simulink model "powerwindow_tl_v04"  (R2020b)
settings: Solver=ode1  StartTime=0.0  StopTime=20.0  FixedStep=0.01  RelTol=1e-3
PreLoadFcn:
  | if exist('tl_preloadfcn','file'), tl_preloadfcn(gcs,'5.1.0.29'); end
PostLoadFcn:
  | if exist('tl_postloadfcn','file'), tl_postloadfcn(gcs,'5.1.0.29'); end
InitFcn:
  | if exist('tlds_init','file'), tlds_init(gcs); end
StartFcn:
  | if exist('tlds_start','file'), tlds_start(gcs); end
StopFcn:
  | if exist('tlds_stop','file'), tlds_stop(gcs); end
undefined symbols (not defined in the file): auto_down_time, auto_up_time, emergency_down_time, position_endstop_top
libraries: tllib x7
(part 2 of 2)

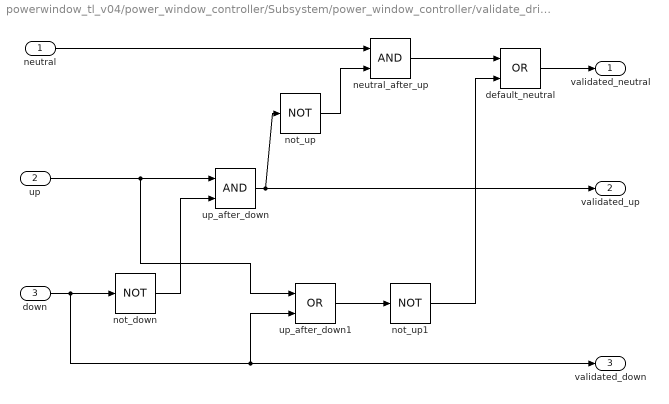
== system powerwindow_tl_v04/power_window_controller/Subsystem/power_window_controller/validate_driver/mutually_exclusive ==
  neutral : Inport  RequirementInfo={} %GIDa_e85989e4_f574_4415_bd99_a29a617e3f19
  up : Inport  RequirementInfo={} %GIDa_79e0b872_de73_4653_8aed_1078f22e8307  Port=2
  down : Inport  RequirementInfo={} %GIDa_e828e409_7827_4f1e_bdb2_ab00d1d51755  Port=3
  default_neutral : Logic  RequirementInfo={} %GIDa_6e7c89da_e8ec_42d0_b277_8441aa3b2da5  Operator=OR  AllPortsSameDT=off  OutDataTypeStr=boolean  mask(TL_LogicalOperator){data={'date',738614.85802565969}}
      settings: CopyFcn=if exist('copy_tlblock','file')==2,copy_tlblock(gcbh);end  DeleteFcn=if exist('delete_tlblock','file')==2,delete_tlblock(gcbh);end  NameChangeFcn=if exist('rename_tlblock','file')==2,rename_tlblock(gcbh);end  OpenFcn=if exist('tl_open_blockdlg','file')==2,tl_open_blockdlg(gcbh);else,open_system(gcbh,'force');end
      mask Help: eval(['if exist(''tl_online_help'',''file'') == 2, tl_online_help(''Topic'',''TL_LogicalOperator''),else, web([''jar:file:///'',matlabroot,''/help/toolbox/simulink/help.jar!/slref/' lower(get_param(gcbh,'Blocktype')) '.html''], ''-helpbrowser''),end'])
      mask Display:
      | [x,y] = tlDrawBrandOnBlockIcon(gcbh);
      | plot(x,y);
  neutral_after_up : Logic  RequirementInfo={} %GIDa_9dd159d3_f1a8_40e9_b9b6_cfadfa6bcd63  AllPortsSameDT=off  OutDataTypeStr=boolean  mask(TL_LogicalOperator){data={'date',738614.85802585643}}
      settings: CopyFcn=if exist('copy_tlblock','file')==2,copy_tlblock(gcbh);end  DeleteFcn=if exist('delete_tlblock','file')==2,delete_tlblock(gcbh);end  NameChangeFcn=if exist('rename_tlblock','file')==2,rename_tlblock(gcbh);end  OpenFcn=if exist('tl_open_blockdlg','file')==2,tl_open_blockdlg(gcbh);else,open_system(gcbh,'force');end
      mask Help: eval(['if exist(''tl_online_help'',''file'') == 2, tl_online_help(''Topic'',''TL_LogicalOperator''),else, web([''jar:file:///'',matlabroot,''/help/toolbox/simulink/help.jar!/slref/' lower(get_param(gcbh,'Blocktype')) '.html''], ''-helpbrowser''),end'])
      mask Display:
      | [x,y] = tlDrawBrandOnBlockIcon(gcbh);
      | plot(x,y);
  not_down : Logic  RequirementInfo={} %GIDa_325b76a6_5f95_47f1_8093_96a77913412f  Operator=NOT  Inputs=1  AllPortsSameDT=off  OutDataTypeStr=boolean  mask(TL_LogicalOperator){data={'date',738614.85802605329}}
      settings: CopyFcn=if exist('copy_tlblock','file')==2,copy_tlblock(gcbh);end  DeleteFcn=if exist('delete_tlblock','file')==2,delete_tlblock(gcbh);end  NameChangeFcn=if exist('rename_tlblock','file')==2,rename_tlblock(gcbh);end  OpenFcn=if exist('tl_open_blockdlg','file')==2,tl_open_blockdlg(gcbh);else,open_system(gcbh,'force');end
      mask Help: eval(['if exist(''tl_online_help'',''file'') == 2, tl_online_help(''Topic'',''TL_LogicalOperator''),else, web([''jar:file:///'',matlabroot,''/help/toolbox/simulink/help.jar!/slref/' lower(get_param(gcbh,'Blocktype')) '.html''], ''-helpbrowser''),end'])
      mask Display:
      | [x,y] = tlDrawBrandOnBlockIcon(gcbh);
      | plot(x,y);
  not_up : Logic  RequirementInfo={} %GIDa_8ed9eef4_b39a_42b2_b85d_a376d662d4ef  Operator=NOT  Inputs=1  AllPortsSameDT=off  OutDataTypeStr=boolean  mask(TL_LogicalOperator){data={'date',738614.85802625003}}
      settings: CopyFcn=if exist('copy_tlblock','file')==2,copy_tlblock(gcbh);end  DeleteFcn=if exist('delete_tlblock','file')==2,delete_tlblock(gcbh);end  NameChangeFcn=if exist('rename_tlblock','file')==2,rename_tlblock(gcbh);end  OpenFcn=if exist('tl_open_blockdlg','file')==2,tl_open_blockdlg(gcbh);else,open_system(gcbh,'force');end
      mask Help: eval(['if exist(''tl_online_help'',''file'') == 2, tl_online_help(''Topic'',''TL_LogicalOperator''),else, web([''jar:file:///'',matlabroot,''/help/toolbox/simulink/help.jar!/slref/' lower(get_param(gcbh,'Blocktype')) '.html''], ''-helpbrowser''),end'])
      mask Display:
      | [x,y] = tlDrawBrandOnBlockIcon(gcbh);
      | plot(x,y);
  not_up1 : Logic  RequirementInfo={} %GIDa_2cd6821b_0d1f_4019_80b4_a85897f079be  Operator=NOT  Inputs=1  AllPortsSameDT=off  OutDataTypeStr=boolean  mask(TL_LogicalOperator){data={'date',738614.8580264583}}
      settings: CopyFcn=if exist('copy_tlblock','file')==2,copy_tlblock(gcbh);end  DeleteFcn=if exist('delete_tlblock','file')==2,delete_tlblock(gcbh);end  NameChangeFcn=if exist('rename_tlblock','file')==2,rename_tlblock(gcbh);end  OpenFcn=if exist('tl_open_blockdlg','file')==2,tl_open_blockdlg(gcbh);else,open_system(gcbh,'force');end
      mask Help: eval(['if exist(''tl_online_help'',''file'') == 2, tl_online_help(''Topic'',''TL_LogicalOperator''),else, web([''jar:file:///'',matlabroot,''/help/toolbox/simulink/help.jar!/slref/' lower(get_param(gcbh,'Blocktype')) '.html''], ''-helpbrowser''),end'])
      mask Display:
      | [x,y] = tlDrawBrandOnBlockIcon(gcbh);
      | plot(x,y);
  up_after_down : Logic  RequirementInfo={} %GIDa_7a4c5de0_0dcd_4b80_97c3_db695de2395f  AllPortsSameDT=off  OutDataTypeStr=boolean  mask(TL_LogicalOperator){data={'date',738614.85802667821}}
      settings: CopyFcn=if exist('copy_tlblock','file')==2,copy_tlblock(gcbh);end  DeleteFcn=if exist('delete_tlblock','file')==2,delete_tlblock(gcbh);end  NameChangeFcn=if exist('rename_tlblock','file')==2,rename_tlblock(gcbh);end  OpenFcn=if exist('tl_open_blockdlg','file')==2,tl_open_blockdlg(gcbh);else,open_system(gcbh,'force');end
      mask Help: eval(['if exist(''tl_online_help'',''file'') == 2, tl_online_help(''Topic'',''TL_LogicalOperator''),else, web([''jar:file:///'',matlabroot,''/help/toolbox/simulink/help.jar!/slref/' lower(get_param(gcbh,'Blocktype')) '.html''], ''-helpbrowser''),end'])
      mask Display:
      | [x,y] = tlDrawBrandOnBlockIcon(gcbh);
      | plot(x,y);
  up_after_down1 : Logic  RequirementInfo={} %GIDa_1f278933_bf51_48e2_9675_d8c687793405  Operator=OR  AllPortsSameDT=off  OutDataTypeStr=boolean  mask(TL_LogicalOperator){data={'date',738614.85802687495}}
      settings: CopyFcn=if exist('copy_tlblock','file')==2,copy_tlblock(gcbh);end  DeleteFcn=if exist('delete_tlblock','file')==2,delete_tlblock(gcbh);end  NameChangeFcn=if exist('rename_tlblock','file')==2,rename_tlblock(gcbh);end  OpenFcn=if exist('tl_open_blockdlg','file')==2,tl_open_blockdlg(gcbh);else,open_system(gcbh,'force');end
      mask Help: eval(['if exist(''tl_online_help'',''file'') == 2, tl_online_help(''Topic'',''TL_LogicalOperator''),else, web([''jar:file:///'',matlabroot,''/help/toolbox/simulink/help.jar!/slref/' lower(get_param(gcbh,'Blocktype')) '.html''], ''-helpbrowser''),end'])
      mask Display:
      | [x,y] = tlDrawBrandOnBlockIcon(gcbh);
      | plot(x,y);
  validated_neutral : Outport  RequirementInfo={} %GIDa_0c6fa346_badf_42ff_932b_e169c438461b
  validated_up : Outport  RequirementInfo={} %GIDa_32e12f58_52d3_40ea_bb48_426aa1e5382d  Port=2
  validated_down : Outport  RequirementInfo={} %GIDa_7a72f20d_c129_4212_af4e_58d14cc49123  Port=3
  wires:
  default_neutral/1 -> validated_neutral/1
  neutral_after_up/1 -> default_neutral/1
  not_up1/1 -> default_neutral/2
  up_after_down1/1 -> not_up1/1
  not_down/1 -> up_after_down/2
  down/1 -> up_after_down1/2, validated_down/1, not_down/1
  up/1 -> up_after_down1/1, up_after_down/1
  up_after_down/1 -> not_up/1, validated_up/1
  not_up/1 -> neutral_after_up/2
  neutral/1 -> neutral_after_up/1

== system powerwindow_tl_v04/power_window_controller/Subsystem/power_window_controller/validate_passenger/check_down ==
  action : Inport  RequirementInfo={} %GIDa_8cd64062_4875_4c08_89a2_40b359a38367
  endstop : Inport  RequirementInfo={} %GIDa_6c5e80aa_8734_491d_9f8c_5569e355bb20  Port=2
  allow_action : Logic  RequirementInfo={} %GIDa_cae1b0df_d7c1_4fdf_9144_dc5ac73a8c8b  AllPortsSameDT=off  OutDataTypeStr=boolean  mask(TL_LogicalOperator){data={'date',738614.85802708333}}
      settings: CopyFcn=if exist('copy_tlblock','file')==2,copy_tlblock(gcbh);end  DeleteFcn=if exist('delete_tlblock','file')==2,delete_tlblock(gcbh);end  NameChangeFcn=if exist('rename_tlblock','file')==2,rename_tlblock(gcbh);end  OpenFcn=if exist('tl_open_blockdlg','file')==2,tl_open_blockdlg(gcbh);else,open_system(gcbh,'force');end
      mask Help: eval(['if exist(''tl_online_help'',''file'') == 2, tl_online_help(''Topic'',''TL_LogicalOperator''),else, web([''jar:file:///'',matlabroot,''/help/toolbox/simulink/help.jar!/slref/' lower(get_param(gcbh,'Blocktype')) '.html''], ''-helpbrowser''),end'])
      mask Display:
      | [x,y] = tlDrawBrandOnBlockIcon(gcbh);
      | plot(x,y);
  not : Logic  RequirementInfo={} %GIDa_81a8c55c_911f_4048_a2e3_38a43e0ac93c  Operator=NOT  Inputs=1  AllPortsSameDT=off  OutDataTypeStr=boolean  mask(TL_LogicalOperator){data={'date',738614.85802730324}}
      settings: CopyFcn=if exist('copy_tlblock','file')==2,copy_tlblock(gcbh);end  DeleteFcn=if exist('delete_tlblock','file')==2,delete_tlblock(gcbh);end  NameChangeFcn=if exist('rename_tlblock','file')==2,rename_tlblock(gcbh);end  OpenFcn=if exist('tl_open_blockdlg','file')==2,tl_open_blockdlg(gcbh);else,open_system(gcbh,'force');end
      mask Help: eval(['if exist(''tl_online_help'',''file'') == 2, tl_online_help(''Topic'',''TL_LogicalOperator''),else, web([''jar:file:///'',matlabroot,''/help/toolbox/simulink/help.jar!/slref/' lower(get_param(gcbh,'Blocktype')) '.html''], ''-helpbrowser''),end'])
      mask Display:
      | [x,y] = tlDrawBrandOnBlockIcon(gcbh);
      | plot(x,y);
  checked_action : Outport  RequirementInfo={} %GIDa_d8e89354_c011_44cf_a51a_50c2da3321e3
  wires:
  action/1 -> allow_action/1
  not/1 -> allow_action/2
  allow_action/1 -> checked_action/1  "checked_action"
  endstop/1 -> not/1

== system powerwindow_tl_v04/power_window_controller/Subsystem/power_window_controller/validate_passenger/check_up ==
  action : Inport  RequirementInfo={} %GIDa_16ed169f_1b1b_4c1c_b5b0_3f0dc41c3f8a
  endstop : Inport  RequirementInfo={} %GIDa_f000520e_93d2_4920_b47a_7f458da2e19a  Port=2
  allow_action : Logic  RequirementInfo={} %GIDa_826e665b_884d_46e0_be0a_702d5d571800  AllPortsSameDT=off  OutDataTypeStr=boolean  mask(TL_LogicalOperator){data={'date',738614.85802752315}}
      settings: CopyFcn=if exist('copy_tlblock','file')==2,copy_tlblock(gcbh);end  DeleteFcn=if exist('delete_tlblock','file')==2,delete_tlblock(gcbh);end  NameChangeFcn=if exist('rename_tlblock','file')==2,rename_tlblock(gcbh);end  OpenFcn=if exist('tl_open_blockdlg','file')==2,tl_open_blockdlg(gcbh);else,open_system(gcbh,'force');end
      mask Help: eval(['if exist(''tl_online_help'',''file'') == 2, tl_online_help(''Topic'',''TL_LogicalOperator''),else, web([''jar:file:///'',matlabroot,''/help/toolbox/simulink/help.jar!/slref/' lower(get_param(gcbh,'Blocktype')) '.html''], ''-helpbrowser''),end'])
      mask Display:
      | [x,y] = tlDrawBrandOnBlockIcon(gcbh);
      | plot(x,y);
  not : Logic  RequirementInfo={} %GIDa_f0e1a078_cc07_48cc_b00b_1e590c6be31e  Operator=NOT  Inputs=1  AllPortsSameDT=off  OutDataTypeStr=boolean  mask(TL_LogicalOperator){data={'date',738614.85802770837}}
      settings: CopyFcn=if exist('copy_tlblock','file')==2,copy_tlblock(gcbh);end  DeleteFcn=if exist('delete_tlblock','file')==2,delete_tlblock(gcbh);end  NameChangeFcn=if exist('rename_tlblock','file')==2,rename_tlblock(gcbh);end  OpenFcn=if exist('tl_open_blockdlg','file')==2,tl_open_blockdlg(gcbh);else,open_system(gcbh,'force');end
      mask Help: eval(['if exist(''tl_online_help'',''file'') == 2, tl_online_help(''Topic'',''TL_LogicalOperator''),else, web([''jar:file:///'',matlabroot,''/help/toolbox/simulink/help.jar!/slref/' lower(get_param(gcbh,'Blocktype')) '.html''], ''-helpbrowser''),end'])
      mask Display:
      | [x,y] = tlDrawBrandOnBlockIcon(gcbh);
      | plot(x,y);
  checked_action : Outport  RequirementInfo={} %GIDa_f36de57c_5397_44fe_9775_f4676f4d6ee7
  wires:
  not/1 -> allow_action/2
  endstop/1 -> not/1
  action/1 -> allow_action/1
  allow_action/1 -> checked_action/1  "checked_action"

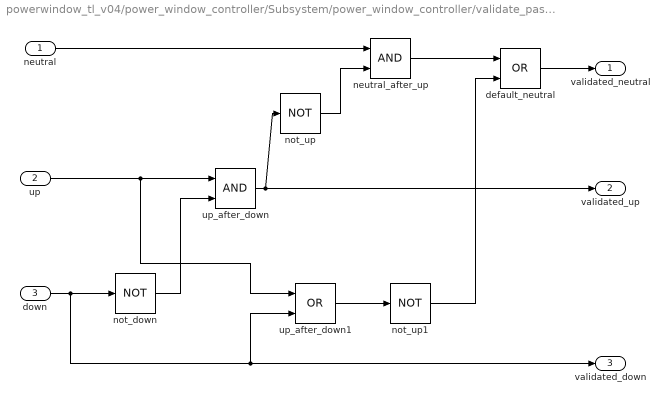
== system powerwindow_tl_v04/power_window_controller/Subsystem/power_window_controller/validate_passenger/mutually_exclusive ==
  neutral : Inport  RequirementInfo={} %GIDa_2277cd25_915f_45f2_802c_d71d72a0241f
  up : Inport  RequirementInfo={} %GIDa_5dd23a3b_b230_464f_b7d2_23423f1a037d  Port=2
  down : Inport  RequirementInfo={} %GIDa_ec6a8333_fae6_4906_9f5b_139dda985102  Port=3
  default_neutral : Logic  RequirementInfo={} %GIDa_c3d63baf_43df_45e4_aeba_3c12a5166081  Operator=OR  AllPortsSameDT=off  OutDataTypeStr=boolean  mask(TL_LogicalOperator){data={'date',738614.85802789347}}
      settings: CopyFcn=if exist('copy_tlblock','file')==2,copy_tlblock(gcbh);end  DeleteFcn=if exist('delete_tlblock','file')==2,delete_tlblock(gcbh);end  NameChangeFcn=if exist('rename_tlblock','file')==2,rename_tlblock(gcbh);end  OpenFcn=if exist('tl_open_blockdlg','file')==2,tl_open_blockdlg(gcbh);else,open_system(gcbh,'force');end
      mask Help: eval(['if exist(''tl_online_help'',''file'') == 2, tl_online_help(''Topic'',''TL_LogicalOperator''),else, web([''jar:file:///'',matlabroot,''/help/toolbox/simulink/help.jar!/slref/' lower(get_param(gcbh,'Blocktype')) '.html''], ''-helpbrowser''),end'])
      mask Display:
      | [x,y] = tlDrawBrandOnBlockIcon(gcbh);
      | plot(x,y);
  neutral_after_up : Logic  RequirementInfo={} %GIDa_ec9809e9_f798_4b3f_b61c_af040d406103  AllPortsSameDT=off  OutDataTypeStr=boolean  mask(TL_LogicalOperator){data={'date',738614.85802810185}}
      settings: CopyFcn=if exist('copy_tlblock','file')==2,copy_tlblock(gcbh);end  DeleteFcn=if exist('delete_tlblock','file')==2,delete_tlblock(gcbh);end  NameChangeFcn=if exist('rename_tlblock','file')==2,rename_tlblock(gcbh);end  OpenFcn=if exist('tl_open_blockdlg','file')==2,tl_open_blockdlg(gcbh);else,open_system(gcbh,'force');end
      mask Help: eval(['if exist(''tl_online_help'',''file'') == 2, tl_online_help(''Topic'',''TL_LogicalOperator''),else, web([''jar:file:///'',matlabroot,''/help/toolbox/simulink/help.jar!/slref/' lower(get_param(gcbh,'Blocktype')) '.html''], ''-helpbrowser''),end'])
      mask Display:
      | [x,y] = tlDrawBrandOnBlockIcon(gcbh);
      | plot(x,y);
  not_down : Logic  RequirementInfo={} %GIDa_62793087_cf19_434f_99ed_e3dcfcfc4ef5  Operator=NOT  Inputs=1  AllPortsSameDT=off  OutDataTypeStr=boolean  mask(TL_LogicalOperator){data={'date',738614.85802829859}}
      settings: CopyFcn=if exist('copy_tlblock','file')==2,copy_tlblock(gcbh);end  DeleteFcn=if exist('delete_tlblock','file')==2,delete_tlblock(gcbh);end  NameChangeFcn=if exist('rename_tlblock','file')==2,rename_tlblock(gcbh);end  OpenFcn=if exist('tl_open_blockdlg','file')==2,tl_open_blockdlg(gcbh);else,open_system(gcbh,'force');end
      mask Help: eval(['if exist(''tl_online_help'',''file'') == 2, tl_online_help(''Topic'',''TL_LogicalOperator''),else, web([''jar:file:///'',matlabroot,''/help/toolbox/simulink/help.jar!/slref/' lower(get_param(gcbh,'Blocktype')) '.html''], ''-helpbrowser''),end'])
      mask Display:
      | [x,y] = tlDrawBrandOnBlockIcon(gcbh);
      | plot(x,y);
  not_up : Logic  RequirementInfo={} %GIDa_e37fd2a9_d4cc_400d_9210_9d34d301a22f  Operator=NOT  Inputs=1  AllPortsSameDT=off  OutDataTypeStr=boolean  mask(TL_LogicalOperator){data={'date',738614.8580285185}}
      settings: CopyFcn=if exist('copy_tlblock','file')==2,copy_tlblock(gcbh);end  DeleteFcn=if exist('delete_tlblock','file')==2,delete_tlblock(gcbh);end  NameChangeFcn=if exist('rename_tlblock','file')==2,rename_tlblock(gcbh);end  OpenFcn=if exist('tl_open_blockdlg','file')==2,tl_open_blockdlg(gcbh);else,open_system(gcbh,'force');end
      mask Help: eval(['if exist(''tl_online_help'',''file'') == 2, tl_online_help(''Topic'',''TL_LogicalOperator''),else, web([''jar:file:///'',matlabroot,''/help/toolbox/simulink/help.jar!/slref/' lower(get_param(gcbh,'Blocktype')) '.html''], ''-helpbrowser''),end'])
      mask Display:
      | [x,y] = tlDrawBrandOnBlockIcon(gcbh);
      | plot(x,y);
  not_up1 : Logic  RequirementInfo={} %GIDa_b3804168_938d_4578_aa76_633e70a2c927  Operator=NOT  Inputs=1  AllPortsSameDT=off  OutDataTypeStr=boolean  mask(TL_LogicalOperator){data={'date',738614.85802871524}}
      settings: CopyFcn=if exist('copy_tlblock','file')==2,copy_tlblock(gcbh);end  DeleteFcn=if exist('delete_tlblock','file')==2,delete_tlblock(gcbh);end  NameChangeFcn=if exist('rename_tlblock','file')==2,rename_tlblock(gcbh);end  OpenFcn=if exist('tl_open_blockdlg','file')==2,tl_open_blockdlg(gcbh);else,open_system(gcbh,'force');end
      mask Help: eval(['if exist(''tl_online_help'',''file'') == 2, tl_online_help(''Topic'',''TL_LogicalOperator''),else, web([''jar:file:///'',matlabroot,''/help/toolbox/simulink/help.jar!/slref/' lower(get_param(gcbh,'Blocktype')) '.html''], ''-helpbrowser''),end'])
      mask Display:
      | [x,y] = tlDrawBrandOnBlockIcon(gcbh);
      | plot(x,y);
  up_after_down : Logic  RequirementInfo={} %GIDa_9c14ace3_0aaa_4433_a4cd_6617714538f0  AllPortsSameDT=off  OutDataTypeStr=boolean  mask(TL_LogicalOperator){data={'date',738614.85802891199}}
      settings: CopyFcn=if exist('copy_tlblock','file')==2,copy_tlblock(gcbh);end  DeleteFcn=if exist('delete_tlblock','file')==2,delete_tlblock(gcbh);end  NameChangeFcn=if exist('rename_tlblock','file')==2,rename_tlblock(gcbh);end  OpenFcn=if exist('tl_open_blockdlg','file')==2,tl_open_blockdlg(gcbh);else,open_system(gcbh,'force');end
      mask Help: eval(['if exist(''tl_online_help'',''file'') == 2, tl_online_help(''Topic'',''TL_LogicalOperator''),else, web([''jar:file:///'',matlabroot,''/help/toolbox/simulink/help.jar!/slref/' lower(get_param(gcbh,'Blocktype')) '.html''], ''-helpbrowser''),end'])
      mask Display:
      | [x,y] = tlDrawBrandOnBlockIcon(gcbh);
      | plot(x,y);
  up_after_down1 : Logic  RequirementInfo={} %GIDa_08faeccd_9450_4183_8177_3d3d98bc27b3  Operator=OR  AllPortsSameDT=off  OutDataTypeStr=boolean  mask(TL_LogicalOperator){data={'date',738614.85802910884}}
      settings: CopyFcn=if exist('copy_tlblock','file')==2,copy_tlblock(gcbh);end  DeleteFcn=if exist('delete_tlblock','file')==2,delete_tlblock(gcbh);end  NameChangeFcn=if exist('rename_tlblock','file')==2,rename_tlblock(gcbh);end  OpenFcn=if exist('tl_open_blockdlg','file')==2,tl_open_blockdlg(gcbh);else,open_system(gcbh,'force');end
      mask Help: eval(['if exist(''tl_online_help'',''file'') == 2, tl_online_help(''Topic'',''TL_LogicalOperator''),else, web([''jar:file:///'',matlabroot,''/help/toolbox/simulink/help.jar!/slref/' lower(get_param(gcbh,'Blocktype')) '.html''], ''-helpbrowser''),end'])
      mask Display:
      | [x,y] = tlDrawBrandOnBlockIcon(gcbh);
      | plot(x,y);
  validated_neutral : Outport  RequirementInfo={} %GIDa_70412c7d_a157_4e94_b5d8_bf29a8a0833a
  validated_up : Outport  RequirementInfo={} %GIDa_a3590772_ff6b_49a9_b818_5f38836f6597  Port=2
  validated_down : Outport  RequirementInfo={} %GIDa_6849a50e_72f0_4401_8aff_7de038e55647  Port=3
  wires:
  default_neutral/1 -> validated_neutral/1
  neutral_after_up/1 -> default_neutral/1
  not_up1/1 -> default_neutral/2
  up_after_down1/1 -> not_up1/1
  not_down/1 -> up_after_down/2
  down/1 -> up_after_down1/2, validated_down/1, not_down/1
  up/1 -> up_after_down1/1, up_after_down/1
  up_after_down/1 -> not_up/1, validated_up/1
  not_up/1 -> neutral_after_up/2
  neutral/1 -> neutral_after_up/1

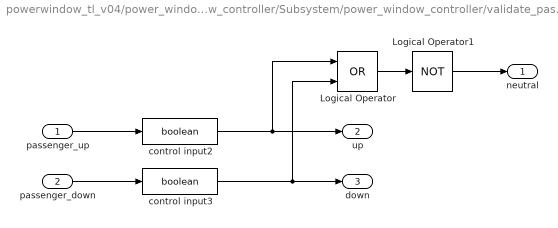
== system powerwindow_tl_v04/power_window_controller/Subsystem/power_window_controller/validate_passenger/passenger_switch ==
  passenger_up : Inport  RequirementInfo={} %GIDa_9ab6ac34_bec8_4376_98db_96cfe725543b
  passenger_down : Inport  RequirementInfo={} %GIDa_0004a635_8eca_422c_82ad_a414e70e7240  Port=2
  Logical Operator : Logic  RequirementInfo={} %GIDa_b8f6f227_f708_4f3d_8b1a_fc5999201240  Operator=OR  AllPortsSameDT=off  OutDataTypeStr=boolean  mask(TL_LogicalOperator){data={'date',738614.85802930559}}
      settings: CopyFcn=if exist('copy_tlblock','file')==2,copy_tlblock(gcbh);end  DeleteFcn=if exist('delete_tlblock','file')==2,delete_tlblock(gcbh);end  NameChangeFcn=if exist('rename_tlblock','file')==2,rename_tlblock(gcbh);end  OpenFcn=if exist('tl_open_blockdlg','file')==2,tl_open_blockdlg(gcbh);else,open_system(gcbh,'force');end
      mask Help: eval(['if exist(''tl_online_help'',''file'') == 2, tl_online_help(''Topic'',''TL_LogicalOperator''),else, web([''jar:file:///'',matlabroot,''/help/toolbox/simulink/help.jar!/slref/' lower(get_param(gcbh,'Blocktype')) '.html''], ''-helpbrowser''),end'])
      mask Display:
      | [x,y] = tlDrawBrandOnBlockIcon(gcbh);
      | plot(x,y);
  Logical Operator1 : Logic  RequirementInfo={} %GIDa_37115b96_8895_4482_9dfe_a04d81c064fe  Operator=NOT  Inputs=1  AllPortsSameDT=off  OutDataTypeStr=boolean  mask(TL_LogicalOperator){data={'date',738614.85802950233}}
      settings: CopyFcn=if exist('copy_tlblock','file')==2,copy_tlblock(gcbh);end  DeleteFcn=if exist('delete_tlblock','file')==2,delete_tlblock(gcbh);end  NameChangeFcn=if exist('rename_tlblock','file')==2,rename_tlblock(gcbh);end  OpenFcn=if exist('tl_open_blockdlg','file')==2,tl_open_blockdlg(gcbh);else,open_system(gcbh,'force');end
      mask Help: eval(['if exist(''tl_online_help'',''file'') == 2, tl_online_help(''Topic'',''TL_LogicalOperator''),else, web([''jar:file:///'',matlabroot,''/help/toolbox/simulink/help.jar!/slref/' lower(get_param(gcbh,'Blocktype')) '.html''], ''-helpbrowser''),end'])
      mask Display:
      | [x,y] = tlDrawBrandOnBlockIcon(gcbh);
      | plot(x,y);
  control input2 : DataTypeConversion  RequirementInfo={} %GIDa_8a46e1bc_7b51_4b42_afe4_fc1c0033716e  OutDataTypeStr=boolean  SaturateOnIntegerOverflow=on  RndMeth=Zero  mask(TL_Rescaler){data={'date',738614.8580335764}}
      settings: CopyFcn=if exist('copy_tlblock','file')==2,copy_tlblock(gcbh);end  DeleteFcn=if exist('delete_tlblock','file')==2,delete_tlblock(gcbh);end  NameChangeFcn=if exist('rename_tlblock','file')==2,rename_tlblock(gcbh);end  OpenFcn=if exist('tl_open_blockdlg','file')==2,tl_open_blockdlg(gcbh);else,open_system(gcbh,'force');end
      mask Help: eval(['if exist(''tl_online_help'',''file'') == 2, tl_online_help(''Topic'',''TL_Rescaler''),else, web([''jar:file:///'',matlabroot,''/help/toolbox/simulink/help.jar!/slref/' lower(get_param(gcbh,'Blocktype')) '.html''], ''-helpbrowser''),end'])
      mask Display:
      | [x,y] = tlDrawBrandOnBlockIcon(gcbh);
      | plot(x,y);
  control input3 : DataTypeConversion  RequirementInfo={} %GIDa_a0d61dcd_05f0_4f70_b8c6_f10cfdf0efe1  OutDataTypeStr=boolean  SaturateOnIntegerOverflow=on  RndMeth=Zero  mask(TL_Rescaler){data={'date',738614.85803380783}}
      settings: CopyFcn=if exist('copy_tlblock','file')==2,copy_tlblock(gcbh);end  DeleteFcn=if exist('delete_tlblock','file')==2,delete_tlblock(gcbh);end  NameChangeFcn=if exist('rename_tlblock','file')==2,rename_tlblock(gcbh);end  OpenFcn=if exist('tl_open_blockdlg','file')==2,tl_open_blockdlg(gcbh);else,open_system(gcbh,'force');end
      mask Help: eval(['if exist(''tl_online_help'',''file'') == 2, tl_online_help(''Topic'',''TL_Rescaler''),else, web([''jar:file:///'',matlabroot,''/help/toolbox/simulink/help.jar!/slref/' lower(get_param(gcbh,'Blocktype')) '.html''], ''-helpbrowser''),end'])
      mask Display:
      | [x,y] = tlDrawBrandOnBlockIcon(gcbh);
      | plot(x,y);
  neutral : Outport  RequirementInfo={} %GIDa_5cbb1afd_1901_468e_aebe_9a6f428f3089
  up : Outport  RequirementInfo={} %GIDa_9371c689_46cb_4e5a_a906_a8fb90d187ee  Port=2
  down : Outport  RequirementInfo={} %GIDa_b1ac157b_14df_46ca_bc0b_91b38617cb83  Port=3
  wires:
  Logical Operator1/1 -> neutral/1
  Logical Operator/1 -> Logical Operator1/1
  control input3/1 -> Logical Operator/2, down/1
  control input2/1 -> Logical Operator/1, up/1
  passenger_down/1 -> control input3/1
  passenger_up/1 -> control input2/1

== stateflow chart powerwindow_tl_v04/power_window_controller/Subsystem/power_window_controller/control ==
  state safe
    state driverNeutral
      entry:
      moveUp = 0;
      moveDown = 0;
      state passengerneutral
        entry:
        moveUp = 0;
        moveDown = 0;
      state passengerDown
        entry: moveDown = 1;
        exit:   moveDown = 0;
        state iniPassengerDown
        state passengerDown
        state autoPassengerDown
        iniPassengerDown -> (junction 14) : after(auto_down_time,tick)
        (junction 14) -> safe.driverNeutral.passengerDown.passengerDown [order 2]
        (junction 14) -> autoPassengerDown [order 1] : [passenger_neutral]
      state passengerUp
        entry: moveUp = 1;
        exit: moveUp = 0;
        state iniPassengerUp
        state PassengerUp
        state autoPassengerUp
        iniPassengerUp -> (junction 29) : after(auto_up_time,tick)
        (junction 29) -> PassengerUp [order 2]
        (junction 29) -> autoPassengerUp [order 1] : [passenger_neutral]
      (default) -> passengerneutral
      passengerneutral -> iniPassengerUp [order 1] : [passenger_up]
      passengerneutral -> iniPassengerDown [order 2] : [passenger_down]
      safe.driverNeutral.passengerDown.passengerDown -> passengerneutral : [passenger_neutral]
      PassengerUp -> passengerneutral : [passenger_neutral]
      safe.driverNeutral.passengerDown -> passengerneutral [order 1] : [endstop_bottom]
      passengerUp -> passengerneutral [order 2] : [endstop_top]
      safe.driverNeutral.passengerDown -> PassengerUp [order 2] : [passenger_up]
      passengerUp -> safe.driverNeutral.passengerDown.passengerDown [order 1] : [passenger_down]
    state driverUp
      entry: moveUp = 1;
      exit: moveUp = 0;
      state iniDriverUp
      state DriverUp
      state autoDriverUp
      iniDriverUp -> (junction 55) : after(auto_up_time,tick)
      (junction 55) -> DriverUp [order 2]
      (junction 55) -> autoDriverUp [order 1] : [driver_neutral]
    state driverDown
      entry: moveDown = 1;
      exit: moveDown = 0;
      state iniDriverDown
      state DriverDown
      state autoDriverDown
      iniDriverDown -> (junction 44) : after(auto_down_time,tick)
      (junction 44) -> DriverDown [order 2]
      (junction 44) -> autoDriverDown [order 1] : [driver_neutral]
    (default) -> driverNeutral
    driverNeutral -> iniDriverDown [order 2] : [driver_down]
    DriverDown -> driverNeutral : [driver_neutral]
    driverDown -> driverNeutral [order 1] : [endstop_bottom]
    DriverUp -> driverNeutral : [driver_neutral]
    driverUp -> driverNeutral [order 2] : [endstop_top]
    driverNeutral -> iniDriverUp [order 1] : [driver_up]
    driverDown -> DriverUp [order 2] : [driver_up]
    driverUp -> DriverDown [order 1] : [driver_down]
  state emergencyDown
    entry:
    moveUp = 0;
    moveDown = 1;
  emergencyDown -> passengerneutral : [endstop_bottom | after(emergency_down_time,tick)]
  (default) -> safe
  safe -> emergencyDown : [obstacle]
  data: auto_up_time input; auto_down_time input; emergency_down_time input; driver_neutral input; driver_up input; driver_down input; passenger_neutral input; passenger_up input; passenger_down input; obstacle input; endstop_bottom input; endstop_top input; moveDown output double; moveUp output
  data auto_up_time settings: description=$TL$ type=UInt8; date=20170127T121847; $TL$
  data auto_down_time settings: description=$TL$ type=UInt8; date=20170127T121847; $TL$
  data emergency_down_time settings: description=$TL$ type=UInt8; date=20170127T121847; $TL$
  data driver_neutral settings: description=$TL$ type=Bool; $TL$
  data driver_up settings: description=$TL$ type=Bool; $TL$
  data driver_down settings: description=$TL$ type=Bool; $TL$
  data passenger_neutral settings: description=$TL$ type=Bool; $TL$
  data passenger_up settings: description=$TL$ type=Bool; $TL$
  data passenger_down settings: description=$TL$ type=Bool; $TL$
  data obstacle settings: description=$TL$ type=Bool; $TL$
  data endstop_bottom settings: description=$TL$ type=Bool; $TL$
  data endstop_top settings: description=$TL$ type=Bool; $TL$
  data moveDown settings: description=$TL$ type=Bool; date=20170127T121852; $TL$
  data moveUp settings: description=$TL$ type=Bool; date=20170127T121852; $TL$
